simulink library "TCDial"  (R2025a)
settings: Solver=VariableStepAuto  StartTime=0.0  StopTime=10.0  RelTol=1e-3
undefined symbols (not defined in the file or in its folder): raptor_xcp_function, StateSignal
libraries: Utilities x4, simulink x4, Raptor_lib x3
settings Model: Creator=serga  LastModifiedBy=hyuga

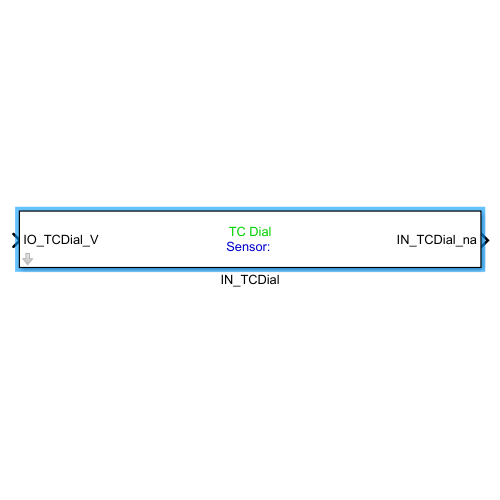
[thumbnail: Simulink's stored preview of the top-level diagram]
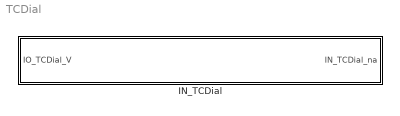
== system TCDial ==
  IN_TCDial : Subsystem  mask{pos=''}
      mask prompts: pos "Position"
      mask Display:
      | color('green')
      | disp('TC Dial\n');
      | color('blue')
      | disp(['\nSensor: ' pos]);
      | color('black')
      | port_label('input', 1, ['IO_TCDial' pos '_V']);
      | port_label('output', 1, ['IN_TCDial' pos '_na']);

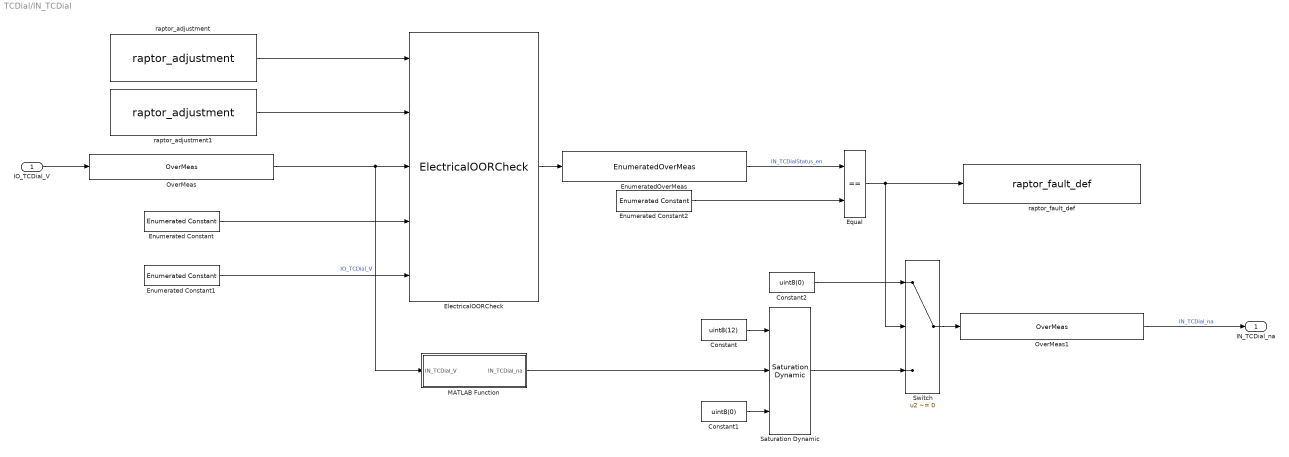
== system TCDial/IN_TCDial ==
  IO_TCDial_V : Inport
  Constant : Constant  Value=uint8(12)
  Constant1 : Constant  Value=uint8(0)
  Constant2 : Constant  Value=uint8(0)
  ElectricalOORCheck : Utilities/ElectricalOORCheck
  Enumerated Constant : simulink/Sources/Enumerated Constant  OutDataTypeStr=Enum: StateSignal  Value=StateSignal.Normal  SampleTime=inf
  Enumerated Constant1 : simulink/Sources/Enumerated Constant  OutDataTypeStr=Enum: StateSignal  Value=StateSignal.Fault  SampleTime=inf
  Enumerated Constant2 : simulink/Sources/Enumerated Constant  OutDataTypeStr=Enum: StateSignal  Value=StateSignal.Fault  SampleTime=inf
  EnumeratedOverMeas : Utilities/EnumeratedOverMeas  sigName=['IN_TCDial' pos 'Status_en']  enumName='StateSignal'
  Equal : RelationalOperator  Operator===  OutDataTypeStr=boolean  RndMeth=Simplest  InputSameDT=off
  MATLAB Function : MATLAB Function  TreatAsAtomicUnit=on
  OverMeas : Utilities/OverMeas  sigName=['IO_TCDial' pos '_V']  minimum=0  maximum=5
  OverMeas1 : Utilities/OverMeas  sigName=['IN_TCDial' pos '_na']  minimum=0  maximum=11
  Saturation Dynamic : simulink/Discontinuities/Saturation Dynamic  OutMin=[]  OutMax=[]  OutDataTypeStr=Inherit: Same as second input  OutDataType=fixdt(1, 16)  OutScaling=2^-10  DoSatur=off
  Switch : Switch  Criteria=u2 ~= 0  SaturateOnIntegerOverflow=off  InputSameDT=off
  raptor_adjustment : Raptor_lib/Data Storage/raptor_adjustment  paramName=['IN_ThrottlePosition' pos 'HighThresh_V']  nameSource=Parameter  initValue=5  dataType=single  storage=Calibration  calDispType=Number  calEnum={'False', 'True'}  calGain=1.0  calOffset=0.0  calMax=5  calMin=0  calFormat='-1'  calUnit=''  calHelp=''  calAccess=1  calFunction=raptor_xcp_function(gcb)  calDispHeaders=off  calColHeaders={'Col1' 'Col2' 'Col3'}  calRowHeaders={'Row1' 'Row2' 'Row3'}
      settings: SourceProductName=Raptor
  raptor_adjustment1 : Raptor_lib/Data Storage/raptor_adjustment  paramName=['IN_ThrottlePosition' pos 'LowThresh_V']  nameSource=Parameter  initValue=0  dataType=single  storage=Calibration  calDispType=Number  calEnum={'False', 'True'}  calGain=1.0  calOffset=0.0  calMax=5  calMin=0  calFormat='-1'  calUnit=''  calHelp=''  calAccess=1  calFunction=raptor_xcp_function(gcb)  calDispHeaders=off  calColHeaders={'Col1' 'Col2' 'Col3'}  calRowHeaders={'Row1' 'Row2' 'Row3'}
      settings: SourceProductName=Raptor
  raptor_fault_def : Raptor_lib/Faults/raptor_fault_def  faultName=['IN_TCDial' pos 'Fault']  persist=off  sticky=off  emisRelated=off  permanent=off  singleTrip=off  clearMethod=Standard  xLimit=25  yLimit=50  calEnable=on  addDisable=off  calAccess=1  calFunction='System | FaultManager'
      settings: SourceProductName=Raptor
  IN_TCDial_na : Outport
  wires:
  IO_TCDial_V/1 -> OverMeas/1
  OverMeas/1 -> MATLAB Function/1(IN_TCDial_V), ElectricalOORCheck/3  "IO_TCDial_V"
  raptor_adjustment/1 -> ElectricalOORCheck/1
  raptor_adjustment1/1 -> ElectricalOORCheck/2
  Enumerated Constant/1 -> ElectricalOORCheck/4
  Enumerated Constant1/1 -> ElectricalOORCheck/5
  ElectricalOORCheck/1 -> EnumeratedOverMeas/1
  Enumerated Constant2/1 -> Equal/2
  Equal/1 -> Switch/2, raptor_fault_def/1
  EnumeratedOverMeas/1 -> Equal/1  "IN_TCDialStatus_en"
  Saturation Dynamic/1 -> Switch/3
  Constant/1 -> Saturation Dynamic/1
  Constant1/1 -> Saturation Dynamic/3
  Constant2/1 -> Switch/1
  OverMeas1/1 -> IN_TCDial_na/1  "IN_TCDial_na"
  Switch/1 -> OverMeas1/1
  MATLAB Function/1(IN_TCDial_na) -> Saturation Dynamic/2

== matlab function TCDial/IN_TCDial/MATLAB Function ==
  data: IN_TCDial_V input; IN_TCDial_na output
function IN_TCDial_na = fcn(IN_TCDial_V)
coder.inline('always')

if ~isscalar(IN_TCDial_V)
    IN_TCDial_na = 0;
    return
end

if (IN_TCDial_V > 4.77) && (IN_TCDial_V <= 5)
    IN_TCDial_na = 0;
elseif (IN_TCDial_V > 4.32) && (IN_TCDial_V <= 4.7)
    IN_TCDial_na = 1;
elseif (IN_TCDial_V > 3.86) && (IN_TCDial_V <= 4.32)
    IN_TCDial_na = 2;
elseif (IN_TCDial_V > 3.41) && (IN_TCDial_V <= 3.86)
    IN_TCDial_na = 3;
elseif (IN_TCDial_V > 2.96) && (IN_TCDial_V <= 3.41)
    IN_TCDial_na = 4;
elseif (IN_TCDial_V > 2.5) && (IN_TCDial_V <= 2.96)
    IN_TCDial_na = 5;
elseif (IN_TCDial_V > 2.05) && (IN_TCDial_V <= 2.5)
    IN_TCDial_na = 6;
elseif (IN_TCDial_V > 1.59) && (IN_TCDial_V <= 2.05)
    IN_TCDial_na = 7;
elseif (IN_TCDial_V > 1.14) && (IN_TCDial_V <= 1.59)
    IN_TCDial_na = 8;
elseif (IN_TCDial_V > 0.68) && (IN_TCDial_V <= 1.14)
    IN_TCDial_na = 9;
elseif (IN_TCDial_V > 0.23) && (IN_TCDial_V <= 0.68)
    IN_TCDial_na = 10;
elseif (IN_TCDial_V > 0) && (IN_TCDial_V <= 0.23)
    IN_TCDial_na = 11;
else
    IN_TCDial_na = 0;
end
